simulink model "AW_test"  (R2015a)
settings: Solver=ode5  StartTime=0.0  StopTime=0.5  FixedStep=1e-5  MaxStep=5e-5  MinStep=1e-14  RelTol=1e-12  AbsTol=1e-12
values from neighbouring files (symbols this model uses):
  Ak = [-315.096994309 -3878.89771101 -17.0292118566 21.2098569883 246.813546014 484.691837637 -149.63417576 -492.819462299 3167.4151908 -130.626932997 -31.9727283183 -412.323742278 ... (144 elements, 12x12)]    [controller.mat]    (also in main_Matlab.m = rlqg.A)
  Ap = A    [main_Matlab.m]    (also in plant.mat = [-12.4193466298 -4275.94904034 0 0 0 0 0 0 0 0 0 0 ... (144 )
  Bk = [-0.00424098668828 0.00299188088287 -0.110971716586 -0.350675357795 -0.314262808957 0.267697856405 -10.0334333049 -9.39488290887 0.852384232314 -56.5067664404 -23.4639342577 -28.187233595]    [controller.mat]    (also in main_Matlab.m = rlqg.B)
  Bp = B    [main_Matlab.m]    (also in plant.mat = [1.07981690619 -1.43007830529 0.100011390918 0.910875595767 )
  Ck = [-247.527908345 97.8275933894 272.025102929 -165.96639153 4.4095489734 -129.340374453 -144.603576366 -212.735555333 46.3002432612 -57.7195976838 55.0038517645 -189.155831414 ... (24 elements, 2x12)]    [controller.mat]    (also in main_Matlab.m = rlqg.C)
  Cp = C    [main_Matlab.m]    (also in plant.mat = [-4.0785585711 1.34396179505 -1.0873585976 -2.76318487234 -1)
  Dk = [0 0]    [controller.mat]    (also in main_Matlab.m = rlqg.D)
  Dp = zeros(1,2)    [main_Matlab.m]    (also in plant.mat = [0 0])
  P = lyap(Ap,Q)    [main_Matlab.m]
undefined symbols (not defined in the file or in its folder): Af, Bf, Cf, Hf
settings Model: Creator=p4wp4w  LastModifiedBy=Ablah

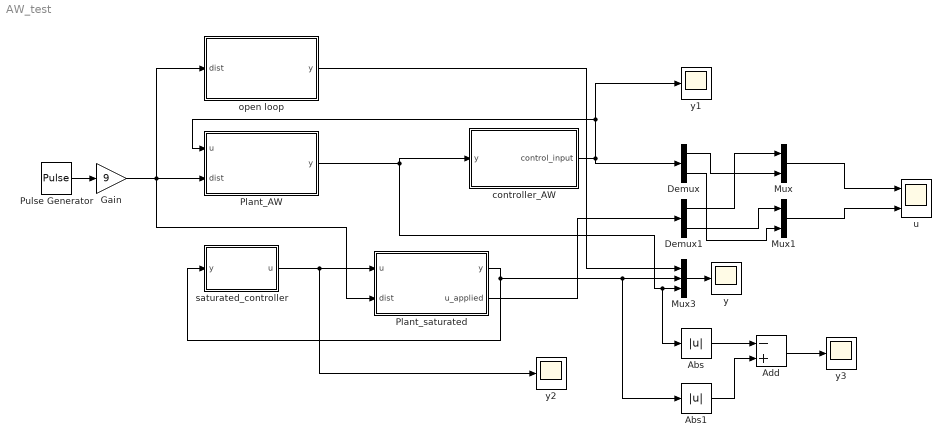
== system AW_test ==
  Abs : Abs
  Abs1 : Abs
  Add : Sum  Inputs=-+
  Demux : Demux  Outputs=2
  Demux1 : Demux  Outputs=2
  Gain : Gain  Gain=9
  Mux : Mux  Inputs=2
  Mux1 : Mux  Inputs=2
  Mux3 : Mux  Inputs=3
  Plant_AW : Subsystem
  Plant_saturated : Subsystem
  Pulse Generator : DiscretePulseGenerator  PulseType=Time based  Period=0.5  PulseWidth=10
  controller_AW : Subsystem
  open loop : Subsystem
  "saturated_controller " : Subsystem
  u : Scope  NumInputPorts=2
      settings: ShowLegends=on  YMin=-0.45~-0.2  YMax=0.2~0.125
  y{,1..3} (4 alike) : Scope
      y settings: ShowLegends=on
      y1 settings: SaveName=ScopeData4
      y2 settings: SaveName=ScopeData6
      y3 settings: ShowLegends=on  SaveName=ScopeData3
  wires:
  Plant_AW/1(y) -> controller_AW/1(y), Abs/1, Mux3/3
  controller_AW/1("control_input ") -> y1/1, Plant_AW/1(u), Demux/1
  Pulse Generator/1 -> Gain/1
  Plant_saturated/1(y) -> Abs1/1, Mux3/2, "saturated_controller "/1(y)
  Demux1/1 -> Mux/1
  Demux/1 -> Mux/2
  Demux1/2 -> Mux1/1
  Demux/2 -> Mux1/2
  Mux/1 -> u/1
  Mux1/1 -> u/2
  Plant_saturated/2(u_applied) -> Demux1/1
  Gain/1 -> Plant_saturated/2(dist), open loop/1(dist), Plant_AW/2(dist)
  open loop/1(y) -> Mux3/1
  Mux3/1 -> y/1
  "saturated_controller "/1(u) -> y2/1, Plant_saturated/1(u)
  Abs/1 -> Add/1
  Abs1/1 -> Add/2
  Add/1 -> y3/1

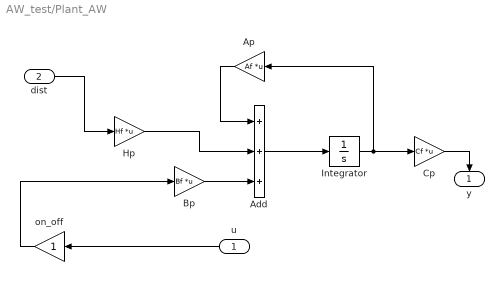
== system AW_test/Plant_AW ==
  u : Inport
  dist : Inport  Port=2
  Add : Sum  Inputs=+++
  Ap : Gain  Gain=Af  Multiplication=Matrix(K*u)
  Bp : Gain  Gain=Bf  Multiplication=Matrix(K*u)
  Cp : Gain  Gain=Cf  Multiplication=Matrix(K*u)
  Hp : Gain  Gain=Hf  Multiplication=Matrix(K*u)
  Integrator : Integrator
  on_off : Gain
  y : Outport
  wires:
  Add/1 -> Integrator/1
  Cp/1 -> y/1
  Hp/1 -> Add/2
  on_off/1 -> Bp/1
  Integrator/1 -> Cp/1, Ap/1
  u/1 -> on_off/1
  Ap/1 -> Add/1
  Bp/1 -> Add/3
  dist/1 -> Hp/1

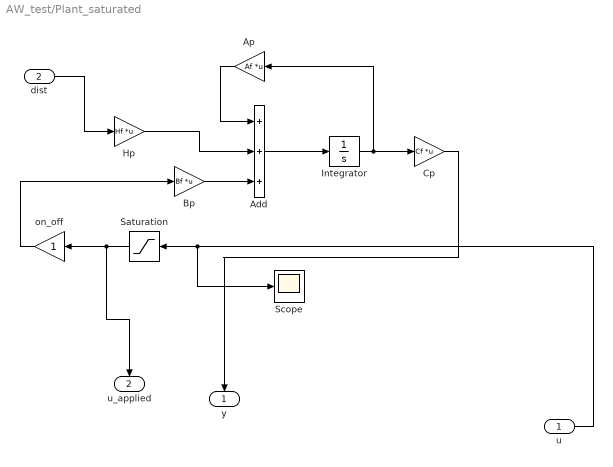
== system AW_test/Plant_saturated ==
  u : Inport
  dist : Inport  Port=2
  Add : Sum  Inputs=+++
  Ap : Gain  Gain=Af  Multiplication=Matrix(K*u)
  Bp : Gain  Gain=Bf  Multiplication=Matrix(K*u)
  Cp : Gain  Gain=Cf  Multiplication=Matrix(K*u)
  Hp : Gain  Gain=Hf  Multiplication=Matrix(K*u)
  Integrator : Integrator
  Saturation : Saturate  UpperLimit=2  LowerLimit=-2
  Scope : Scope
      settings: YMin=-10  YMax=10  SaveName=ScopeData2
  on_off : Gain
  y : Outport
  u_applied : Outport  Port=2
  wires:
  dist/1 -> Hp/1
  Bp/1 -> Add/3
  u/1 -> Scope/1, Saturation/1
  Ap/1 -> Add/1
  Saturation/1 -> u_applied/1, on_off/1
  Integrator/1 -> Ap/1, Cp/1
  on_off/1 -> Bp/1
  Hp/1 -> Add/2
  Cp/1 -> y/1
  Add/1 -> Integrator/1

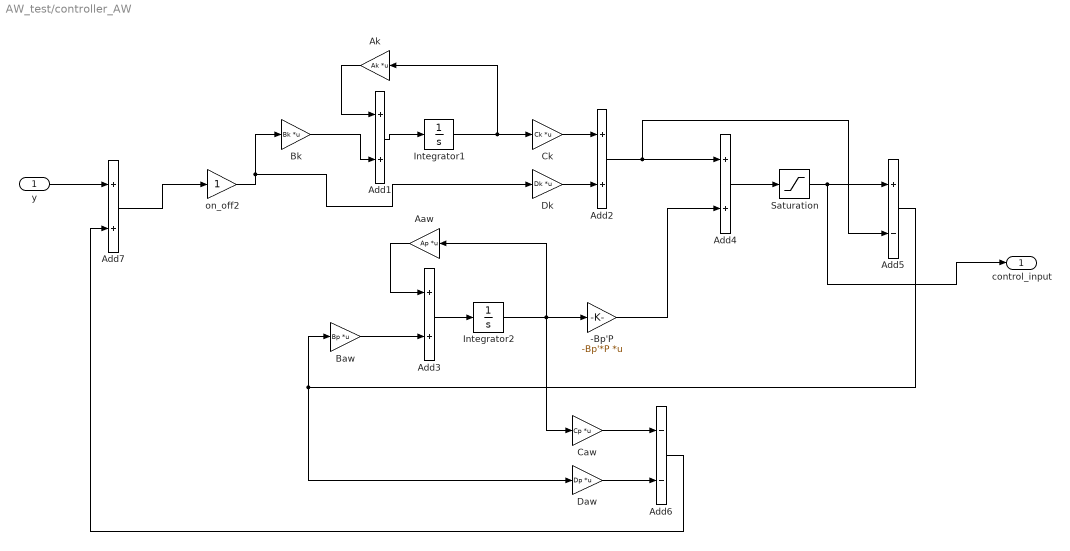
== system AW_test/controller_AW ==
  y : Inport
  -Bp'P : Gain  Gain=-Bp'*P  Multiplication=Matrix(K*u)
  Aaw : Gain  Gain=Ap  Multiplication=Matrix(K*u)
  Add{1..4,7} (5 alike) : Sum
  Add5 : Sum  Inputs=+-
  Add6 : Sum  Inputs=--
  Ak : Gain  Gain=Ak  Multiplication=Matrix(K*u)
  Baw : Gain  Gain=Bp  Multiplication=Matrix(K*u)
  Bk : Gain  Gain=Bk  Multiplication=Matrix(K*u)
  Caw : Gain  Gain=Cp  Multiplication=Matrix(K*u)
  Ck : Gain  Gain=Ck  Multiplication=Matrix(K*u)
  Daw : Gain  Gain=Dp  Multiplication=Matrix(K*u)
  Dk : Gain  Gain=Dk  Multiplication=Matrix(K*u)
  Integrator1 : Integrator
  Integrator2 : Integrator
  Saturation : Saturate  UpperLimit=2  LowerLimit=-2
  on_off2 : Gain
  "control_input " : Outport
  wires:
  Ck/1 -> Add2/1
  Add1/1 -> Integrator1/1
  Ak/1 -> Add1/1
  Bk/1 -> Add1/2
  Integrator1/1 -> Ck/1, Ak/1
  Dk/1 -> Add2/2
  on_off2/1 -> Dk/1, Bk/1
  Add3/1 -> Integrator2/1
  Aaw/1 -> Add3/1
  Baw/1 -> Add3/2
  Integrator2/1 -> Caw/1, -Bp'P/1, Aaw/1
  Add2/1 -> Add5/2, Add4/1
  -Bp'P/1 -> Add4/2
  Add4/1 -> Saturation/1
  Saturation/1 -> "control_input "/1, Add5/1
  Add5/1 -> Daw/1, Baw/1
  Caw/1 -> Add6/1
  Daw/1 -> Add6/2
  y/1 -> Add7/1
  Add7/1 -> on_off2/1
  Add6/1 -> Add7/2

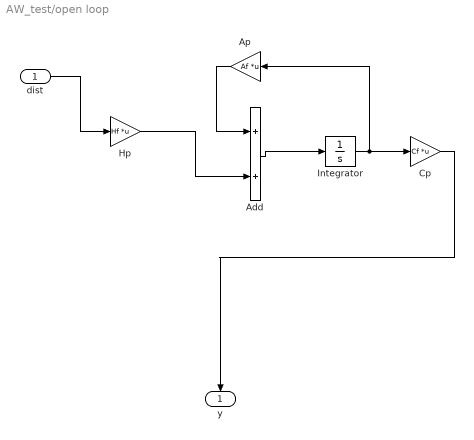
== system AW_test/open loop ==
  dist : Inport
  Add : Sum
  Ap : Gain  Gain=Af  Multiplication=Matrix(K*u)
  Cp : Gain  Gain=Cf  Multiplication=Matrix(K*u)
  Hp : Gain  Gain=Hf  Multiplication=Matrix(K*u)
  Integrator : Integrator
  y : Outport
  wires:
  dist/1 -> Hp/1
  Ap/1 -> Add/1
  Integrator/1 -> Ap/1, Cp/1
  Hp/1 -> Add/2
  Cp/1 -> y/1
  Add/1 -> Integrator/1

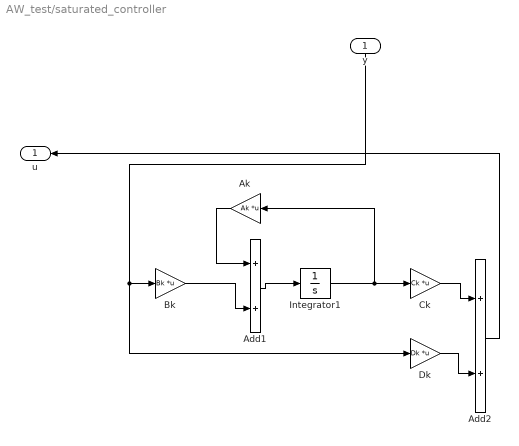
== system AW_test/saturated_controller  ==
  y : Inport
  Add1 : Sum
  Add2 : Sum
  Ak : Gain  Gain=Ak  Multiplication=Matrix(K*u)
  Bk : Gain  Gain=Bk  Multiplication=Matrix(K*u)
  Ck : Gain  Gain=Ck  Multiplication=Matrix(K*u)
  Dk : Gain  Gain=Dk  Multiplication=Matrix(K*u)
  Integrator1 : Integrator
  u : Outport
  wires:
  Bk/1 -> Add1/2
  Add1/1 -> Integrator1/1
  Ck/1 -> Add2/1
  Dk/1 -> Add2/2
  Integrator1/1 -> Ck/1, Ak/1
  Add2/1 -> u/1
  Ak/1 -> Add1/1
  y/1 -> Bk/1, Dk/1
